simulink model "CiEngine"  (R2018a)
settings: Solver=VariableStepAuto  StartTime=0.0  StopTime=inf  RelTol=1e-3  EnableMultiTasking=on
model workspace (MAT data in the model file):
  AccPwrbp = [0 2]
  AccSpdbp = [300 750]
  TimeCnstECP = 0.125
  TimeCnstEGR = 0.125
  TimeCnstETC = 0.085
  TimeCnstICP = 0.125
  TimeCnstIVL = 0.125
  TimeCnstMFA = 0.125
  TimeCnstSWVA = 0.125
  TimeCnstVCR = 0.125
  TimeCnstVGT = 0.15
  TimeCnstVIRL = 0.125
  TimeCnstWGA = 0.15
libraries: autolibutils x1
settings Model: ModifiedByFormat=The MathWorks, Inc.  Creator=The MathWorks, Inc.  LastModifiedBy=The MathWorks, Inc.
settings DataIOCC: DSMLogging=off
settings DebuggingCC: ModelReferenceExtraNoncontSigs=none
settings CodeAppCC: StateflowObjectComments=on
settings GRTTargetCC: TargetLangStandard=C89/C90 (ANSI)
settings ConfigComp: CovMetricSettings=dsw  CovHtmlReporting=on  CovSaveCumulativeToWorkspaceVar=on  CovSaveSingleToWorkspaceVar=on  CovShowResultsExplorer=off  CovExternalEMLEnable=off
settings SimscapeCC: SimscapeNormalizeSystem=off  SimscapeNominalValues={1, 'bar'; 1, 'cm^3/s'; 1, 'bar*kg/s'; 1, 'kJ/kg'; 1, 'kW'; };

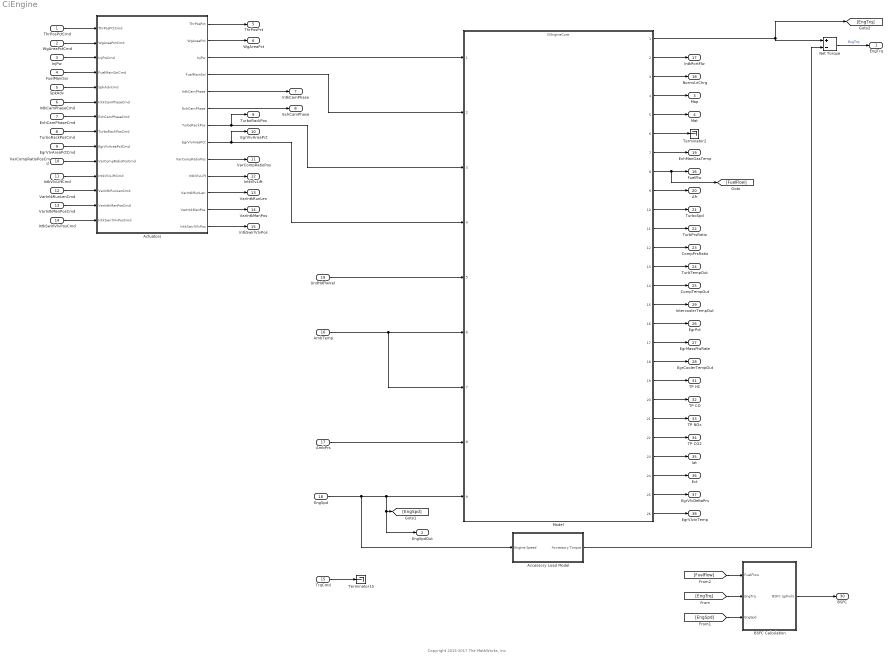
== system CiEngine ==
  note: Copyright 2015-2017 The MathWorks, Inc.
  ThrPosPctCmd : Inport
  WgAreaPctCmd : Inport  Port=2
  InjPw : Inport  Port=3
  FuelMainSoi : Inport  Port=4
  SpkAdv : Inport  Port=5
  IntkCamPhaseCmd : Inport  Port=6
  ExhCamPhaseCmd : Inport  Port=7
  TurboRackPosCmd : Inport  Port=8
  EgrVlvAreaPctCmd : Inport  Port=9
  VarCompRatioPosCmd : Inport  Port=10
  IntkVlvLiftCmd : Inport  Port=11
  VarIntkRunLenCmd : Inport  Port=12
  VarIntkManPosCmd : Inport  Port=13
  IntkSwirlVlvPosCmd : Inport  Port=14
  TrqCmd : Inport  Port=15  Unit=N*m
  AmbTemp : Inport  Port=16
  AmbPrs : Inport  Port=17
  EngSpd : Inport  Port=18  Interpolate=off
  UndHdFlwVel : Inport  Port=19
  Accessory Load Model : Subsystem
  Actuators : Subsystem
  BSFC Calculation : Subsystem
  Model : ModelReference  ModelNameDialog=CiEngineCore  SimulationMode=Normal  ModelReferenceVersion=1.394
  Net Torque : Sum  Inputs=+-
  Terminator15 : Terminator
  Terminator2 : Terminator
  EngTrq : Outport  Unit=N*m
  EngSpdOut : Outport  Port=2
  Map : Outport  Port=3
  Mat : Outport  Port=4
  ThrPosPct : Outport  Port=5
  WgAreaPct : Outport  Port=6
  IntkCamPhase : Outport  Port=7
  ExhCamPhase : Outport  Port=8
  TurboRackPos : Outport  Port=9
  EgrVlvAreaPct : Outport  Port=10
  VarCompRatioPos : Outport  Port=11
  IntkVlvLift : Outport  Port=12
  VarIntkRunLen : Outport  Port=13
  VarIntkManPos : Outport  Port=14
  IntkSwirlVlvPos : Outport  Port=15
  FuelFlw : Outport  Port=16
  IntkPortFlw : Outport  Port=17
  NormAirChrg : Outport  Port=18
  ExhManGasTemp : Outport  Port=19
  Afr : Outport  Port=20
  TurboSpd : Outport  Port=21
  TurbPrsRatio : Outport  Port=22
  CompPrsRatio : Outport  Port=23
  TurbTempOut : Outport  Port=24
  CompTempOut : Outport  Port=25
  EgrPct : Outport  Port=26
  EgrMassFlwRate : Outport  Port=27
  EgrCoolerTempOut : Outport  Port=28
  IntercoolerTempOut : Outport  Port=29
  BSFC : Outport  Port=30  Unit=g/(kW*hr)
  TP HC : Outport  Port=31
  TP CO : Outport  Port=32
  TP NOx : Outport  Port=33
  TP CO2 : Outport  Port=34
  Iat : Outport  Port=35
  Ect : Outport  Port=36
  EgrVlvDeltaPrs : Outport  Port=37
  EgrVlvInTemp : Outport  Port=38
  wires:
  EngSpd/1 -> Model/9, EngSpdOut/1, [EngSpd], Accessory Load Model/1(Engine Speed)
  Model/1 -> [EngTrq], Net Torque/1
  Accessory Load Model/1(Accessory Torque) -> Net Torque/2
  Net Torque/1 -> EngTrq/1  "EngTrq"
  TrqCmd/1 -> Terminator15/1
  [FuelFlow] -> BSFC Calculation/1(FuelFlow)
  [EngTrq] -> BSFC Calculation/2(EngTrq)
  [EngSpd] -> BSFC Calculation/3(EngSpd)
  BSFC Calculation/1(BSFC (g/Kwh)) -> BSFC/1
  Model/8 -> FuelFlw/1, [FuelFlow]
  AmbTemp/1 -> Model/6, Model/7
  Actuators/1(ThrPosPct) -> ThrPosPct/1
  Actuators/2(WgAreaPct) -> WgAreaPct/1
  AmbPrs/1 -> Model/8
  UndHdFlwVel/1 -> Model/5
  Actuators/3(InjPw) -> Model/1
  Actuators/4(FuelMainSoi) -> Model/2
  Actuators/7(TurboRackPos) -> TurboRackPos/1, Model/3
  Actuators/8(EgrVlvAreaPct) -> EgrVlvAreaPct/1, Model/4
  Actuators/5(IntkCamPhase) -> IntkCamPhase/1
  Actuators/6(ExhCamPhase) -> ExhCamPhase/1
  Actuators/9(VarCompRatioPos) -> VarCompRatioPos/1
  Actuators/10(IntkVlvLift) -> IntkVlvLift/1
  Actuators/13(IntkSwirlVlvPos) -> IntkSwirlVlvPos/1
  Actuators/12(VarIntkManPos) -> VarIntkManPos/1
  Actuators/11(VarIntkRunLen) -> VarIntkRunLen/1
  ThrPosPctCmd/1 -> Actuators/1(ThrPosPctCmd)
  WgAreaPctCmd/1 -> Actuators/2(WgAreaPctCmd)
  InjPw/1 -> Actuators/3(InjPwCmd)
  FuelMainSoi/1 -> Actuators/4(FuelMainSoiCmd)
  SpkAdv/1 -> Actuators/5(SpkAdvCmd)
  IntkCamPhaseCmd/1 -> Actuators/6(IntkCamPhaseCmd)
  ExhCamPhaseCmd/1 -> Actuators/7(ExhCamPhaseCmd)
  TurboRackPosCmd/1 -> Actuators/8(TurboRackPosCmd)
  EgrVlvAreaPctCmd/1 -> Actuators/9(EgrVlvAreaPctCmd)
  VarCompRatioPosCmd/1 -> Actuators/10(VarCompRatioPosCmd)
  IntkVlvLiftCmd/1 -> Actuators/11(IntkVlvLiftCmd)
  VarIntkRunLenCmd/1 -> Actuators/12(VarIntkRunLenCmd)
  VarIntkManPosCmd/1 -> Actuators/13(VarIntkManPosCmd)
  IntkSwirlVlvPosCmd/1 -> Actuators/14(IntkSwirlVlvPosCmd)
  Model/2 -> IntkPortFlw/1
  Model/3 -> NormAirChrg/1
  Model/4 -> Map/1
  Model/5 -> Mat/1
  Model/7 -> ExhManGasTemp/1
  Model/6 -> Terminator2/1
  Model/9 -> Afr/1
  Model/10 -> TurboSpd/1
  Model/11 -> TurbPrsRatio/1
  Model/12 -> CompPrsRatio/1
  Model/13 -> TurbTempOut/1
  Model/14 -> CompTempOut/1
  Model/15 -> IntercoolerTempOut/1
  Model/16 -> EgrPct/1
  Model/17 -> EgrMassFlwRate/1
  Model/18 -> EgrCoolerTempOut/1
  Model/19 -> TP HC/1
  Model/20 -> TP CO/1
  Model/21 -> TP NOx/1
  Model/22 -> TP CO2/1
  Model/24 -> Ect/1
  Model/25 -> EgrVlvDeltaPrs/1
  Model/26 -> EgrVlvInTemp/1
  Model/23 -> Iat/1

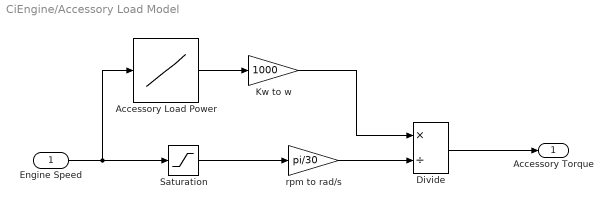
== system CiEngine/Accessory Load Model ==
  Engine Speed : Inport
  Accessory Load Power : Lookup_n-D  NumberOfTableDimensions=1  LookupTableObject=''  BreakpointsForDimension1=AccSpdbp  Table=AccPwrbp  ExtrapMethod=Clip  InternalRulePriority=Speed  RndMeth=Simplest  InputSameDT=on
  Divide : Product  Inputs=*/
  Kw to w : Gain  Gain=1000
  Saturation : Saturate  UpperLimit=Inf  LowerLimit=300
  rpm to rad/s : Gain  Gain=pi/30
  Accessory Torque : Outport
  wires:
  Divide/1 -> Accessory Torque/1
  Accessory Load Power/1 -> Kw to w/1
  Engine Speed/1 -> Accessory Load Power/1, Saturation/1
  Saturation/1 -> rpm to rad/s/1
  rpm to rad/s/1 -> Divide/2
  Kw to w/1 -> Divide/1

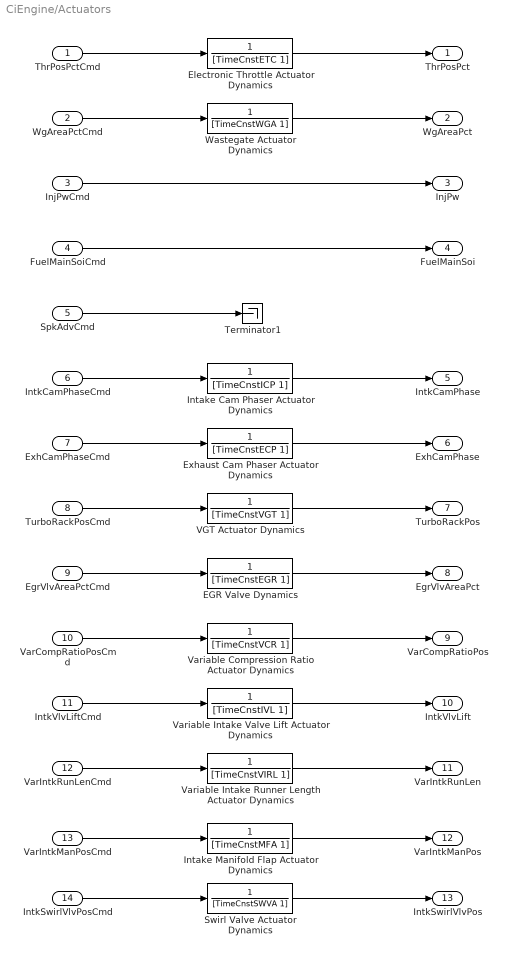
== system CiEngine/Actuators ==
  ThrPosPctCmd : Inport  Unit=%
  WgAreaPctCmd : Inport  Port=2  Unit=%
  InjPwCmd : Inport  Port=3  Unit=ms
  FuelMainSoiCmd : Inport  Port=4  Unit=deg
  SpkAdvCmd : Inport  Port=5  Unit=deg
  IntkCamPhaseCmd : Inport  Port=6  Unit=deg
  ExhCamPhaseCmd : Inport  Port=7  Unit=deg
  TurboRackPosCmd : Inport  Port=8  Unit=1
  EgrVlvAreaPctCmd : Inport  Port=9  Unit=%
  VarCompRatioPosCmd : Inport  Port=10
  IntkVlvLiftCmd : Inport  Port=11
  VarIntkRunLenCmd : Inport  Port=12
  VarIntkManPosCmd : Inport  Port=13
  IntkSwirlVlvPosCmd : Inport  Port=14
  EGR Valve Dynamics : TransferFcn  Denominator=[TimeCnstEGR 1]
  Electronic Throttle Actuator Dynamics : TransferFcn  Denominator=[TimeCnstETC 1]
  Exhaust Cam Phaser Actuator Dynamics : TransferFcn  Denominator=[TimeCnstECP 1]
  Intake Cam Phaser Actuator Dynamics : TransferFcn  Denominator=[TimeCnstICP 1]
  Intake Manifold Flap Actuator Dynamics : TransferFcn  Denominator=[TimeCnstMFA 1]
  Swirl Valve Actuator Dynamics : TransferFcn  Denominator=[TimeCnstSWVA 1]
  Terminator1 : Terminator
  VGT Actuator Dynamics : TransferFcn  Denominator=[TimeCnstVGT 1]
  Variable Compression Ratio Actuator Dynamics : TransferFcn  Denominator=[TimeCnstVCR 1]
  Variable Intake Runner Length Actuator Dynamics : TransferFcn  Denominator=[TimeCnstVIRL 1]
  Variable Intake Valve Lift Actuator Dynamics : TransferFcn  Denominator=[TimeCnstIVL 1]
  Wastegate Actuator Dynamics : TransferFcn  Denominator=[TimeCnstWGA 1]
  ThrPosPct : Outport  Unit=%
  WgAreaPct : Outport  Port=2  Unit=%
  InjPw : Outport  Port=3
  FuelMainSoi : Outport  Port=4
  IntkCamPhase : Outport  Port=5  Unit=deg
  ExhCamPhase : Outport  Port=6  Unit=deg
  TurboRackPos : Outport  Port=7  Unit=1
  EgrVlvAreaPct : Outport  Port=8  Unit=%
  VarCompRatioPos : Outport  Port=9
  IntkVlvLift : Outport  Port=10
  VarIntkRunLen : Outport  Port=11
  VarIntkManPos : Outport  Port=12
  IntkSwirlVlvPos : Outport  Port=13
  wires:
  Variable Compression Ratio Actuator Dynamics/1 -> VarCompRatioPos/1
  Variable Intake Valve Lift Actuator Dynamics/1 -> IntkVlvLift/1
  Variable Intake Runner Length Actuator Dynamics/1 -> VarIntkRunLen/1
  Intake Manifold Flap Actuator Dynamics/1 -> VarIntkManPos/1
  Swirl Valve Actuator Dynamics/1 -> IntkSwirlVlvPos/1
  Intake Cam Phaser Actuator Dynamics/1 -> IntkCamPhase/1
  Exhaust Cam Phaser Actuator Dynamics/1 -> ExhCamPhase/1
  Wastegate Actuator Dynamics/1 -> WgAreaPct/1
  Electronic Throttle Actuator Dynamics/1 -> ThrPosPct/1
  FuelMainSoiCmd/1 -> FuelMainSoi/1
  IntkVlvLiftCmd/1 -> Variable Intake Valve Lift Actuator Dynamics/1
  IntkSwirlVlvPosCmd/1 -> Swirl Valve Actuator Dynamics/1
  WgAreaPctCmd/1 -> Wastegate Actuator Dynamics/1
  ThrPosPctCmd/1 -> Electronic Throttle Actuator Dynamics/1
  ExhCamPhaseCmd/1 -> Exhaust Cam Phaser Actuator Dynamics/1
  IntkCamPhaseCmd/1 -> Intake Cam Phaser Actuator Dynamics/1
  VarIntkManPosCmd/1 -> Intake Manifold Flap Actuator Dynamics/1
  VarCompRatioPosCmd/1 -> Variable Compression Ratio Actuator Dynamics/1
  VarIntkRunLenCmd/1 -> Variable Intake Runner Length Actuator Dynamics/1
  InjPwCmd/1 -> InjPw/1
  VGT Actuator Dynamics/1 -> TurboRackPos/1
  EGR Valve Dynamics/1 -> EgrVlvAreaPct/1
  TurboRackPosCmd/1 -> VGT Actuator Dynamics/1
  EgrVlvAreaPctCmd/1 -> EGR Valve Dynamics/1
  SpkAdvCmd/1 -> Terminator1/1

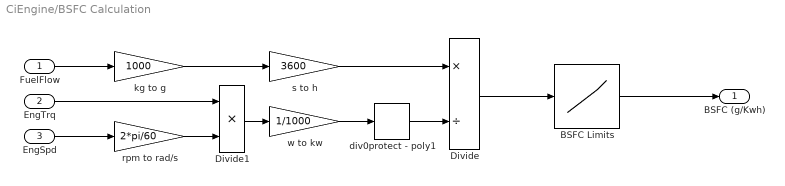
== system CiEngine/BSFC Calculation ==
  FuelFlow : Inport
  EngTrq : Inport  Port=2
  EngSpd : Inport  Port=3
  BSFC Limits : Lookup_n-D  NumberOfTableDimensions=1  BreakpointsForDimension1=[0 500]  Table=[0 500]  ExtrapMethod=Clip  InternalRulePriority=Speed  RndMeth=Simplest  InputSameDT=on
  Divide : Product  Inputs=*/
  Divide1 : Product  Inputs=**
  div0protect - poly1 : autolibutils/div0protect - poly  thresh=1e-6  aMode=aMode
      settings: SourceProductName=Powertrain Blockset  SourceProductBaseCode=PW
  kg to g : Gain  Gain=1000
  rpm to rad/s : Gain  Gain=2*pi/60
  s to h : Gain  Gain=3600
  w to kw : Gain  Gain=1/1000
  BSFC (g/Kwh) : Outport
  wires:
  Divide1/1 -> w to kw/1
  kg to g/1 -> s to h/1
  FuelFlow/1 -> kg to g/1
  rpm to rad/s/1 -> Divide1/2
  EngSpd/1 -> rpm to rad/s/1
  EngTrq/1 -> Divide1/1
  Divide/1 -> BSFC Limits/1
  w to kw/1 -> div0protect - poly1/1
  s to h/1 -> Divide/1
  BSFC Limits/1 -> BSFC (g/Kwh)/1
  div0protect - poly1/1 -> Divide/2
